simulink model "btl_final"  (R2023a)
settings: Solver=VariableStepAuto  StartTime=0.0  StopTime=10  RelTol=1e-3
values from neighbouring files (symbols this model uses):
  Kd = Kp*Td    (= 7.36860974567)    [znpid.m]
  Ki = Kp/Ti    (= 4136.53941578)    [znpid.m]
  Kp = 1.2*T2/T1/K    (= 349.173565165)    [znpid.m]
libraries: simulink x1
settings Model: Creator=adm  LastModifiedBy=Thu
settings RTWCC: GPUComputeCapability=5.0

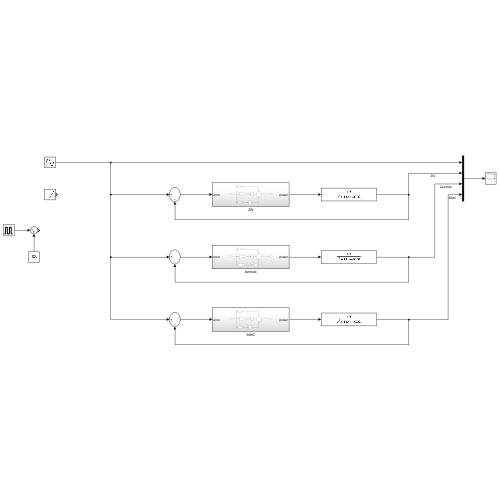
[thumbnail: Simulink's stored preview of the top-level diagram]
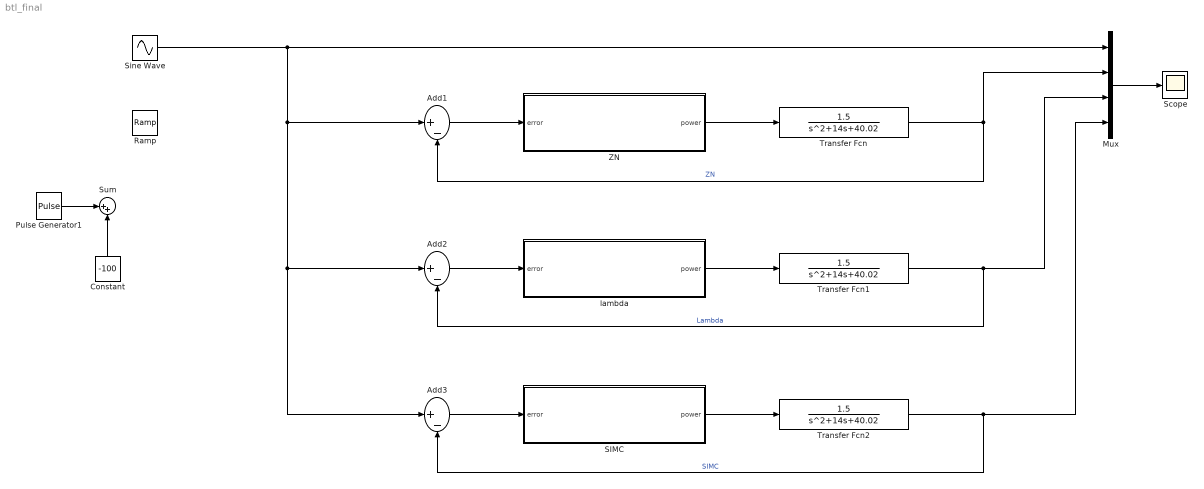
== system btl_final ==
  Add1 : Sum  Inputs=|+-
  Add2 : Sum  Inputs=|+-
  Add3 : Sum  Inputs=|+-
  Constant : Constant  Value=-100
  Mux : Mux
  Pulse Generator1 : DiscretePulseGenerator  PulseType=Time based  Amplitude=200  Period=10  PulseWidth=50
  Ramp : simulink/Sources/Ramp  slope=1  start=0  InitialOutput=0
  SIMC : Subsystem
  Scope : Scope
  Sine Wave : Sin  SampleTime=0
  Sum : Sum  Inputs=|++
  Transfer Fcn : TransferFcn  Numerator=[1.5]  Denominator=[1 14 40.02]
  Transfer Fcn1 : TransferFcn  Numerator=[1.5]  Denominator=[1 14 40.02]
  Transfer Fcn2 : TransferFcn  Numerator=[1.5]  Denominator=[1 14 40.02]
  ZN : Subsystem
  lambda : Subsystem
  wires:
  Transfer Fcn/1 -> Mux/2, Add1/2  "ZN"
  ZN/1(power) -> Transfer Fcn/1
  Add1/1 -> ZN/1(error)
  Mux/1 -> Scope/1
  Transfer Fcn1/1 -> Mux/3, Add2/2  "Lambda"
  Add2/1 -> lambda/1(error)
  lambda/1(power) -> Transfer Fcn1/1
  Transfer Fcn2/1 -> Mux/4, Add3/2  "SIMC"
  Add3/1 -> SIMC/1(error)
  SIMC/1(power) -> Transfer Fcn2/1
  Sine Wave/1 -> Add2/1, Add3/1, Add1/1, Mux/1
  Constant/1 -> Sum/2
  Pulse Generator1/1 -> Sum/1

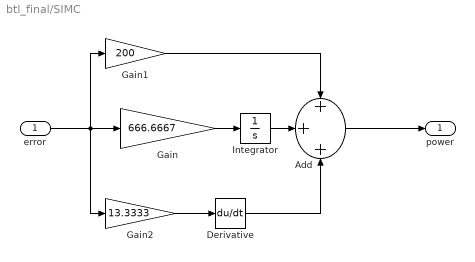
== system btl_final/SIMC ==
  error : Inport
  Add : Sum  Inputs=+++
  Derivative : Derivative
  Gain : Gain  Gain=666.6667
  Gain1 : Gain  Gain=200
  Gain2 : Gain  Gain=13.3333
  Integrator : Integrator
  power : Outport
  wires:
  Add/1 -> power/1
  Derivative/1 -> Add/3
  Gain2/1 -> Derivative/1
  error/1 -> Gain2/1, Gain/1, Gain1/1
  Integrator/1 -> Add/2
  Gain/1 -> Integrator/1
  Gain1/1 -> Add/1

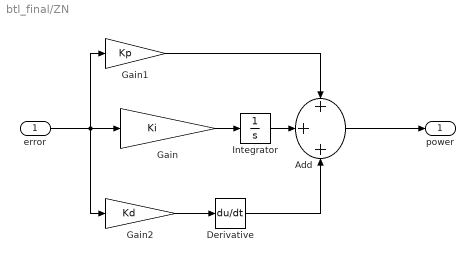
== system btl_final/ZN ==
  error : Inport
  Add : Sum  Inputs=+++
  Derivative : Derivative
  Gain : Gain  Gain=Ki
  Gain1 : Gain  Gain=Kp
  Gain2 : Gain  Gain=Kd
  Integrator : Integrator
  power : Outport
  wires:
  Add/1 -> power/1
  Derivative/1 -> Add/3
  Gain2/1 -> Derivative/1
  error/1 -> Gain2/1, Gain/1, Gain1/1
  Integrator/1 -> Add/2
  Gain/1 -> Integrator/1
  Gain1/1 -> Add/1

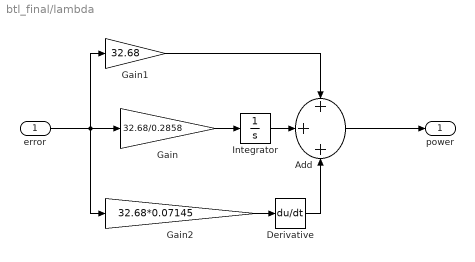
== system btl_final/lambda ==
  error : Inport
  Add : Sum  Inputs=+++
  Derivative : Derivative
  Gain : Gain  Gain=32.68/0.2858
  Gain1 : Gain  Gain=32.68
  Gain2 : Gain  Gain=32.68*0.07145
  Integrator : Integrator
  power : Outport
  wires:
  Add/1 -> power/1
  Derivative/1 -> Add/3
  Gain2/1 -> Derivative/1
  error/1 -> Gain2/1, Gain/1, Gain1/1
  Integrator/1 -> Add/2
  Gain/1 -> Integrator/1
  Gain1/1 -> Add/1
